simulink model "Cap2_Ex1"  (R2021b)
settings: Solver=VariableStepAuto  StartTime=0.0  StopTime=10.0  RelTol=1e-3
settings Model: Creator=Pedro Lamego  LastModifiedBy=Pedro Lamego

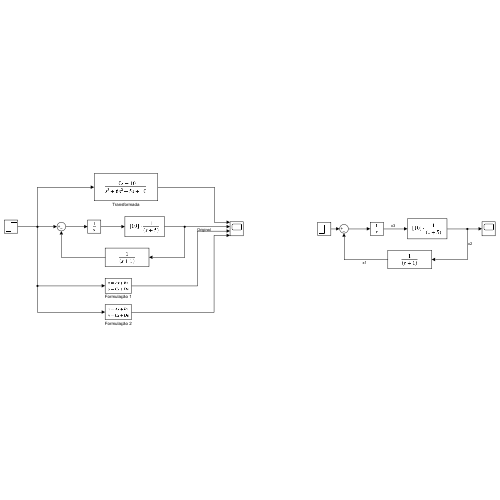
[thumbnail: Simulink's stored preview of the top-level diagram]
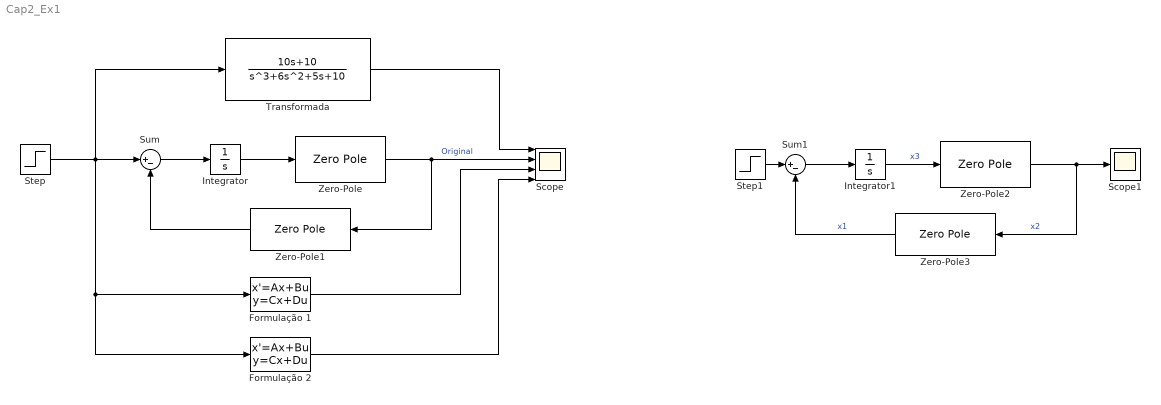
== system Cap2_Ex1 ==
  Formulação 1 : StateSpace  A=[0 1 0; 0 0 1;-10 -5 -6]  B=[0; 10;-50]  C=[1 0 0]  D=[0]  InitialCondition=0
  Formulação 2 : StateSpace  A=[-1 1 0; 0 -5 10;-1 0 0]  B=[0; 0;1]  C=[0 1 0]  D=[0]  InitialCondition=0
  Integrator : Integrator
  Integrator1 : Integrator
  Scope : Scope  NumInputPorts=4
  Scope1 : Scope
  Step : Step  SampleTime=0
  Step1 : Step  SampleTime=0
  Sum : Sum  Inputs=|+-
  Sum1 : Sum  Inputs=|+-
  "Transformada " : TransferFcn  Numerator=[10 10]  Denominator=[1 6 5 10]
  Zero-Pole : ZeroPole  Zeros=[]  Poles=[-5]  Gain=[10]
  Zero-Pole1 : ZeroPole  Zeros=[]  Poles=[-1]
  Zero-Pole2 : ZeroPole  Zeros=[]  Poles=[-5]  Gain=[10]
  Zero-Pole3 : ZeroPole  Zeros=[]  Poles=[-1]
  wires:
  Step1/1 -> Sum1/1
  Formulação 2/1 -> Scope/4
  Integrator1/1 -> Zero-Pole2/1  "x3"
  Zero-Pole2/1 -> Zero-Pole3/1, Scope1/1  "x2"
  Zero-Pole1/1 -> Sum/2
  Step/1 -> Formulação 2/1, Formulação 1/1, "Transformada "/1, Sum/1
  Sum1/1 -> Integrator1/1
  Zero-Pole/1 -> Zero-Pole1/1, Scope/2  "Original"
  Formulação 1/1 -> Scope/3
  Sum/1 -> Integrator/1
  "Transformada "/1 -> Scope/1
  Zero-Pole3/1 -> Sum1/2  "x1"
  Integrator/1 -> Zero-Pole/1
